simulink model "sampleModel1608"  (R2023a)
settings: Solver=VariableStepAuto  StartTime=0.0  StopTime=10.0  RelTol=1e-3
libraries: hdlsllib x2, simulink x1
settings Model: Creator=user1  LastModifiedBy=user1

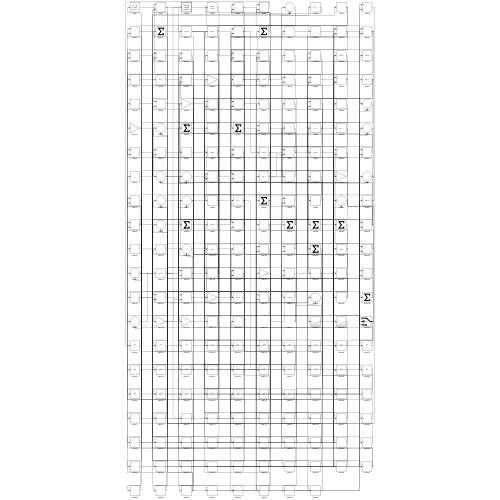
[thumbnail: Simulink's stored preview of the top-level diagram]
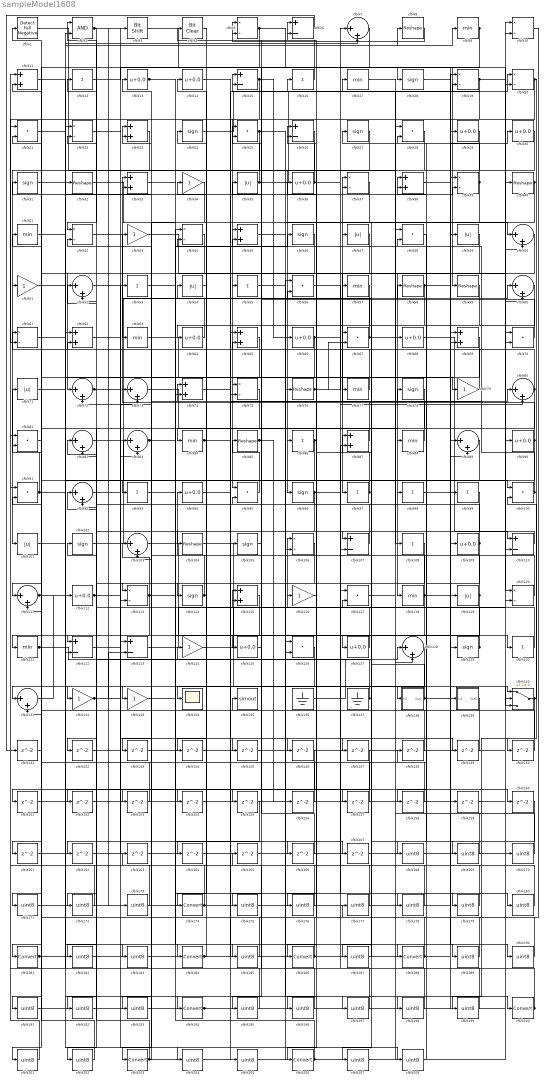
== system sampleModel1608 ==
  cfblk1 : hdlsllib/Logic and Bit Operations/Detect Fall Negative  vinit=0  OutDataTypeStr=boolean
  cfblk{5,10,19..20,22,37,39,42,44,61,75,106,113,120} (14 alike) : Product  Inputs=*/  RndMeth=Zero  SaturateOnIntegerOverflow=on
  cfblk{21,25,28,48,56,67,70,81,91,95,100,117,126} (13 alike) : DotProduct  OutDataTypeStr=Inherit: Inherit via internal rule
  cfblk{35,47,49,54,71,101,119} (7 alike) : Abs  SaturateOnIntegerOverflow=off
  cfblk{18,24,27,31,46,78,96,102,105,114,129} (11 alike) : Signum
  cfblk{7,50,52,60,72..73,80,82..83,89,92,103,111,128,131} (15 alike) : Sum  Inputs=|++
  cfblk{8,32,40,58..59,76,85,104} (8 alike) : Reshape
  cfblk{6,15,26,107,110,122..123} (7 alike) : Sum  Inputs=+-
  cfblk{12,16,53,55,86,93,97..99,108,130} (11 alike) : Sum  Inputs=+
  cfblk{13..14,29..30,36,64,66,68,90,94,109,112,125,127} (14 alike) : Bias  Bias=0.0  SaturateOnIntegerOverflow=off
  cfblk{11,23,33,38,45,62,65,69,74,87,115} (11 alike) : Sum
  cfblk{34,43,51,79,116,124,132..133} (8 alike) : Gain
  cfblk{9,17,41,57,63,77,84,88,118,121} (10 alike) : MinMax
  cfblk134 : Scope
  cfblk135 : ToWorkspace  VariableName=simout  SaveFormat=Timeseries  SampleTime=-1
  cfblk136 : Ground
  cfblk137 : Ground
  cfblk138 : Subsystem
      settings: LibrarySourceBlock=|
      | hdlsllib/Ports &
      | Subsystems/Subsystem
  cfblk139 : Subsystem
      settings: LibrarySourceBlock=|
      | hdlsllib/Ports &
      | Subsystems/Subsystem
  cfblk140 : Switch  SaturateOnIntegerOverflow=off  InputSameDT=off
  cfblk{141..167} (27 alike) : Delay  SampleTime=1
  cfblk{168..173,175..180,182..183,185,187,189..193,195..199,201..202,204..205,207..208} (32 alike) : DataTypeConversion  OutDataTypeStr=uint8  SaturateOnIntegerOverflow=off  RndMeth=Floor
  cfblk{174,181,184,186,188,194,200,203,206} (9 alike) : DataTypeConversion  SaturateOnIntegerOverflow=off  RndMeth=Floor
  cfblk2 : Logic  AllPortsSameDT=off  OutDataTypeStr=boolean
  cfblk3 : hdlsllib/Logic and Bit Operations/Bit Shift  mode=Shift Left Logical  N=0
  cfblk4 : simulink/Logic and Bit Operations/Bit Clear  iBit=0
      settings: LibrarySourceBlock=|
      | hdlsllib/Logic and Bit
      | Operations/Bit Clear
  wires:
  cfblk78/1 -> cfblk118/1
  cfblk29/1 -> cfblk95/1
  cfblk47/1 -> cfblk97/1
  cfblk95/1 -> cfblk85/1
  cfblk20/1 -> cfblk55/1, cfblk150/1
  cfblk23/1 -> cfblk101/1
  cfblk46/1 -> cfblk72/1
  cfblk15/1 -> cfblk45/1, cfblk66/1
  cfblk101/1 -> cfblk32/1
  cfblk59/1 -> cfblk122/1
  cfblk50/1 -> cfblk98/1
  cfblk1/1 -> cfblk108/1
  cfblk131/1 -> cfblk112/1
  cfblk26/1 -> cfblk96/1
  cfblk90/1 -> cfblk33/1, cfblk196/1
  cfblk65/1 -> cfblk75/1
  cfblk99/1 -> cfblk174/1
  cfblk103/1 -> cfblk127/1
  cfblk9/1 -> cfblk59/1, cfblk111/2
  cfblk100/1 -> cfblk74/1, cfblk73/1, cfblk44/2
  cfblk113/1 -> cfblk103/1, cfblk142/1, cfblk166/1
  cfblk41/1 -> cfblk184/1
  cfblk8/1 -> cfblk5/1
  cfblk60/1 -> cfblk114/1
  cfblk73/1 -> cfblk88/1
  cfblk102/1 -> cfblk58/1
  cfblk111/1 -> cfblk8/1, cfblk153/1
  cfblk87/1 -> cfblk61/1
  cfblk114/1 -> cfblk94/1, cfblk72/2, cfblk42/2
  cfblk120/1 -> cfblk87/1
  cfblk94/1 -> cfblk80/1
  cfblk17/1 -> cfblk68/1
  cfblk28/1 -> cfblk206/1
  cfblk83/1 -> cfblk133/1, cfblk130/1
  cfblk68/1 -> cfblk110/1
  cfblk129/1 -> cfblk54/1, cfblk82/1
  cfblk132/1 -> cfblk123/2, cfblk73/2
  cfblk85/1 -> cfblk155/1, cfblk156/1
  cfblk42/1 -> cfblk63/1
  cfblk63/1 -> cfblk139/1(In1)
  cfblk64/1 -> cfblk43/1
  cfblk108/1 -> cfblk132/1
  cfblk84/1 -> cfblk38/2, cfblk164/1
  cfblk130/1 -> cfblk62/2
  cfblk139/1(Out1) -> cfblk135/1
  cfblk35/1 -> cfblk17/1, cfblk25/1, cfblk77/1
  cfblk109/1 -> cfblk2/1, cfblk158/1
  cfblk127/1 -> cfblk106/1
  cfblk54/1 -> cfblk14/1
  cfblk19/1 -> cfblk120/1, cfblk15/2, cfblk61/2
  cfblk97/1 -> cfblk93/1, cfblk26/2
  cfblk121/1 -> cfblk128/1, cfblk37/2
  cfblk118/1 -> cfblk140/3, cfblk31/1, cfblk172/1, cfblk175/1
  cfblk13/1 -> cfblk138/1(In1), cfblk125/1, cfblk167/1
  cfblk107/1 -> cfblk6/1
  cfblk86/1 -> cfblk122/2, cfblk36/1
  cfblk39/1 -> cfblk27/1, cfblk104/1
  cfblk34/1 -> cfblk113/1
  cfblk115/1 -> cfblk121/1
  cfblk3/1 -> cfblk129/1
  cfblk76/1 -> cfblk7/1, cfblk67/2
  cfblk31/1 -> cfblk7/2
  cfblk71/1 -> cfblk79/1
  cfblk138/1(Out1) -> cfblk19/1, cfblk117/2
  cfblk52/1 -> cfblk188/1
  cfblk128/1 -> cfblk131/1
  cfblk37/1 -> cfblk134/1
  cfblk16/1 -> cfblk4/1
  cfblk117/1 -> cfblk39/2
  cfblk93/1 -> cfblk46/1
  cfblk22/1 -> cfblk194/1
  cfblk96/1 -> cfblk140/1, cfblk152/1
  cfblk66/1 -> cfblk84/1, cfblk80/2
  cfblk82/1 -> cfblk109/1
  cfblk137/1 -> cfblk34/1, cfblk92/2
  cfblk5/1 -> cfblk20/2, cfblk154/1
  cfblk21/1 -> cfblk200/1
  cfblk74/1 -> cfblk20/1
  cfblk104/1 -> cfblk140/2
  cfblk123/1 -> cfblk115/1
  cfblk124/1 -> cfblk10/1
  cfblk112/1 -> cfblk53/1, cfblk3/1, cfblk173/1
  cfblk32/1 -> cfblk74/2
  cfblk98/1 -> cfblk30/1
  cfblk43/1 -> cfblk110/2
  cfblk119/1 -> cfblk5/2, cfblk23/2, cfblk161/1, cfblk162/1
  cfblk89/1 -> cfblk181/1
  cfblk72/1 -> cfblk83/2, cfblk145/1
  cfblk25/1 -> cfblk64/1, cfblk50/1
  cfblk30/1 -> cfblk113/2
  cfblk70/1 -> cfblk15/1
  cfblk49/1 -> cfblk86/1
  cfblk91/1 -> cfblk71/1, cfblk100/1
  cfblk105/1 -> cfblk35/1
  cfblk57/1 -> cfblk186/1
  cfblk136/1 -> cfblk19/2
  cfblk27/1 -> cfblk51/1
  cfblk110/1 -> cfblk107/1
  cfblk40/1 -> cfblk67/1, cfblk143/1
  cfblk77/1 -> cfblk23/1
  cfblk88/1 -> cfblk37/1
  cfblk36/1 -> cfblk26/1, cfblk9/1
  cfblk58/1 -> cfblk49/1, cfblk38/1, cfblk187/1
  cfblk80/1 -> cfblk47/1, cfblk111/1
  cfblk79/1 -> cfblk12/1
  cfblk126/1 -> cfblk203/1
  cfblk125/1 -> cfblk95/2
  cfblk140/1 -> cfblk100/2, cfblk169/1
  cfblk67/1 -> cfblk33/2, cfblk60/1
  cfblk12/1 -> cfblk18/1
  cfblk24/1 -> cfblk16/1
  cfblk2/1 -> cfblk42/1, cfblk157/1
  cfblk6/1 -> cfblk141/1
  cfblk141/1 -> cfblk1/1
  cfblk142/1 -> cfblk123/1
  cfblk143/1 -> cfblk10/2
  cfblk4/1 -> cfblk144/1
  cfblk145/1 -> cfblk45/2
  cfblk133/1 -> cfblk146/1
  cfblk122/1 -> cfblk147/1
  cfblk148/1 -> cfblk91/2
  cfblk55/1 -> cfblk149/1
  cfblk149/1 -> cfblk39/1
  cfblk150/1 -> cfblk103/2
  cfblk44/1 -> cfblk151/1
  cfblk151/1 -> cfblk87/2
  cfblk152/1 -> cfblk60/2
  cfblk153/1 -> cfblk62/1
  cfblk154/1 -> cfblk106/2
  cfblk156/1 -> cfblk25/2
  cfblk157/1 -> cfblk131/2
  cfblk158/1 -> cfblk65/2
  cfblk38/1 -> cfblk159/1
  cfblk92/1 -> cfblk160/1
  cfblk161/1 -> cfblk83/1
  cfblk162/1 -> cfblk70/2
  cfblk163/1 -> cfblk50/2
  cfblk165/1 -> cfblk120/2
  cfblk166/1 -> cfblk115/2
  cfblk167/1 -> cfblk128/2
  cfblk48/1 -> cfblk168/1
  cfblk168/1 -> cfblk148/1
  cfblk169/1 -> cfblk48/1
  cfblk170/1 -> cfblk48/2
  cfblk81/1 -> cfblk171/1
  cfblk171/1 -> cfblk76/1
  cfblk172/1 -> cfblk81/1
  cfblk173/1 -> cfblk81/2
  cfblk174/1 -> cfblk75/2, cfblk91/1
  cfblk175/1 -> cfblk99/1
  cfblk116/1 -> cfblk176/1
  cfblk176/1 -> cfblk13/1
  cfblk10/1 -> cfblk177/1
  cfblk177/1 -> cfblk116/1
  cfblk56/1 -> cfblk178/1
  cfblk178/1 -> cfblk124/1
  cfblk144/1 -> cfblk179/1
  cfblk179/1 -> cfblk56/1
  cfblk53/1 -> cfblk180/1
  cfblk180/1 -> cfblk56/2
  cfblk181/1 -> cfblk2/2, cfblk105/1
  cfblk155/1 -> cfblk182/1
  cfblk182/1 -> cfblk89/1
  cfblk61/1 -> cfblk183/1
  cfblk183/1 -> cfblk89/2
  cfblk184/1 -> cfblk107/2, cfblk24/1
  cfblk33/1 -> cfblk185/1
  cfblk185/1 -> cfblk41/1
  cfblk186/1 -> cfblk82/2, cfblk29/1
  cfblk187/1 -> cfblk57/1
  cfblk188/1 -> cfblk65/1, cfblk6/2
  cfblk164/1 -> cfblk189/1
  cfblk189/1 -> cfblk52/1
  cfblk18/1 -> cfblk190/1
  cfblk190/1 -> cfblk52/2
  cfblk69/1 -> cfblk191/1
  cfblk191/1 -> cfblk70/1
  cfblk75/1 -> cfblk192/1
  cfblk192/1 -> cfblk69/1
  cfblk147/1 -> cfblk193/1
  cfblk193/1 -> cfblk69/2
  cfblk194/1 -> cfblk170/1, cfblk119/1
  cfblk7/1 -> cfblk195/1
  cfblk195/1 -> cfblk22/1
  cfblk196/1 -> cfblk22/2
  cfblk11/1 -> cfblk197/1
  cfblk197/1 -> cfblk117/1
  cfblk45/1 -> cfblk198/1
  cfblk198/1 -> cfblk11/1
  cfblk159/1 -> cfblk199/1
  cfblk199/1 -> cfblk11/2
  cfblk200/1 -> cfblk165/1, cfblk78/1
  cfblk146/1 -> cfblk201/1
  cfblk201/1 -> cfblk21/1
  cfblk106/1 -> cfblk202/1
  cfblk202/1 -> cfblk21/2
  cfblk203/1 -> cfblk163/1, cfblk90/1, cfblk92/1, cfblk102/1
  cfblk62/1 -> cfblk204/1
  cfblk204/1 -> cfblk126/1
  cfblk14/1 -> cfblk205/1
  cfblk205/1 -> cfblk126/2
  cfblk206/1 -> cfblk44/1, cfblk40/1
  cfblk160/1 -> cfblk207/1
  cfblk207/1 -> cfblk28/1
  cfblk51/1 -> cfblk208/1
  cfblk208/1 -> cfblk28/2

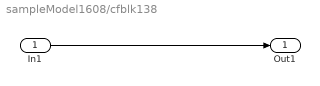
== system sampleModel1608/cfblk138 ==
  In1 : Inport
  Out1 : Outport
  wires:
  In1/1 -> Out1/1

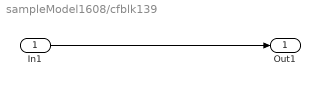
== system sampleModel1608/cfblk139 ==
  In1 : Inport
  Out1 : Outport
  wires:
  In1/1 -> Out1/1
